simulink model "Noa_Nofusion_angle"  (R2020b)
settings: Solver=FixedStepDiscrete  StartTime=0.0  StopTime=Inf  FixedStep=0.01  RelTol=1e-3
PostLoadFcn:
  | if any(exist('dsrtsu_mdlpostloadfcn', 'file') ~= 0), dsrtsu_mdlpostloadfcn('Execute', bdroot); end
InitFcn:
  | , if any(exist('rtifpga_mdlclblib', 'file') ~= 0), rtifpga_mdlclblib('Init', bdroot); end,
  | , if any(exist('dsmpb_private', 'file') ~= 0), dsmpb_private('dsmpb_mdlclblib', 'Init', bdroot); end,
undefined symbols (not defined in the file): ACC_TimeGap_DecSetSwt, ACC_TimeGap_IncSetSwt, AccelPedalPosn, AccelPedalPosnVldty, AccelPedlPosnDiagc, AccPedalOverride, ACU_ShiftInProgress, ADAS_Posn_CurLane, AESSwtReq, ALC_SwtReq, BrkPedalSts, CC_ACC_CANCEL_OFFSwt, CC_ACC_CRUISE_OFFSwt, CC_ACC_DecSetSpd_SetSwt, CC_ACC_IncSetSpd_ResuSwt, CC_ACCSwtErr, CharSpd_ms, CSA_NODE, CURRENT_GEAR, CurrentGearValid, DiscIntNeverNeededParam, DrvDoorSts, DrvSBR, DrvTrqReqOvld, ECMACCInterface, ECMRespACC, ELKSwtReq, EngLimpHomeSts, EngSpd, EngState, EngState_PHEV, EngTrqMaxActSpd, EngTrqMinAct, EPS_DrvInpTrqVal_HighReslolution, EPS_FailSts, EPS_LKATorqOvrlDlvd, EPS_LKATorqOvrlDlvdVld, EPS_LKATrqOvlDlvdSts, EPS_SteerMod, EPS_TrqSnsrSts, EQ4_APPINFO, EQ4_LA_ELEM, EQ4_LA_HDR, EQ4_LAP_ELEM, EQ4_LAP_HDR, EQ4_LH_ELEM, EQ4_LH_HDR, EQ4_LRE_ELEM, EQ4_LRE_HDR, ESS_PedSwtReq, ESS_VehSwtReq, FFogLmpSts_F_Pbox, FLWheelDriveDirection, FLWheelSpd, FrntWiprSwtSts, FrntWshrSwtSts, FRWheelDriveDirection, FRWheelSpd, HazardLmpSwtSts, HCU_AccelPedalPosn_Diag ... (+151)
libraries: simulink x138, dsmpblib x33, canfdmsglib x10
(part 3 of 17)

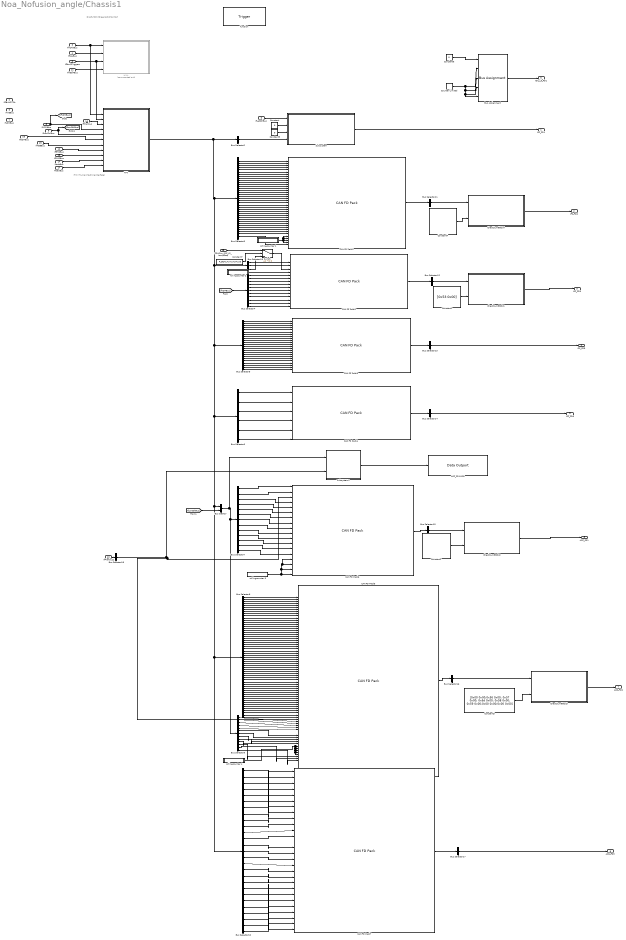
== system Noa_Nofusion_angle/Chassis1 ==
  note: DIAG-MON
      | (DiagnosticMonitor)
  note: HMI
      | (HumanMachineInterface)
  IfFaultTriggers : Inport
  IfFaultDTCs : Inport  Port=2
  IfVCANBus : Inport  Port=3  OutDataTypeStr=Bus: VCAN_BUS
  IfCALBus : Inport  Port=4
  IfVIEBus : Inport  Port=5
  IfVSMBus : Inport  Port=6
  IfLSMBus : Inport  Port=7
  IfLonCtrlBus : Inport  Port=8
  IfLatCtrlBus : Inport  Port=9
  IfPlanbus : Inport  Port=10
  IfVEQ4Bus : Inport  Port=11
  IfEHRBus : Inport  Port=12
  IfDMSBus : Inport  Port=13
  LaneBus : Inport  Port=14
  IfAEBBus : Inport  Port=15
  IfOSMBus : Inport  Port=16
  RoadBus : Inport  Port=17
  CSASim_IDC_L2_LampReq : Inport  Port=18
  function : TriggerPort  TriggerType=function-call  VariantControl=Variant
  ACC_FD1MSG : dsmpblib/Data Outport  Priority=-10000
      settings: SourceProductName=dSPACE Model Interface Blockset
  Bus Assignment : BusAssignment  AssignedSignals=RollingCounter_IDC_L3_1,RollingCounter_IDC_L3_3,RollingCounter_IDC_L3_5,RollingCounter_IDC_L3_4
  Bus Creator : BusCreator  Inputs=2
  Bus Selector10 : BusSelector  OutputSignals=HMI_ACC_FD4.ACCTgtObjAx,HMI_ACC_FD4.ACCTgtObjAy,HMI_ACC_FD4.ACCTgtObjCntAlive,HMI_ACC_FD4.ACCTgtObjDx,HMI_ACC_FD4.ACCTgtObjDy,HMI_ACC_FD4.ACCTgtObjExist,HMI_ACC_FD4.ACCTgtObjID,HMI_ACC_FD4.ACCTgtObjObstcl,HMI_ACC_FD4.ACCTgtObjState,HMI_ACC_FD4.ACCTgtObjVideoCfmd,HMI_ACC_FD4.ACCTgtObjVx,HMI_ACC_FD4.ACCTgtObjVy,HMI_ACC_FD4.ACC_SOSReq,HMI_ACC_FD4.BrdgDst,HMI_ACC_FD4.CurveDst,HMI_ACC_FD4.DrvgOnHiWay,HMI_ACC_FD4.DrvgOnRiLane,HMI_ACC_FD4.DrvrSts,HMI_ACC_FD4.HandsoffDetd,HMI_ACC_FD4.MapDataValid,HMI_ACC_FD4.NavSpdLimUnit,HMI_ACC_FD4.RampDst,HMI_ACC_FD4.RoadCrvt,HMI_ACC_FD4.RoadCrvtFar,HMI_ACC_FD4.SpdLimit,HMI_ACC_FD4.SpdLimitDst,HMI_ACC_FD4.TunnelDst
  Bus Selector{11..17} (7 alike) : BusSelector  OutputSignals=Data
  Bus Selector18 : BusSelector  OutputSignals=PLAN_Longctrl_DecelToStopReq
  Bus Selector19 : BusSelector  OutputSignals=HMI_IFC_FD3.IDC_L2_EmgyLightReq,HMI_IFC_FD3.IDC_L2_FWiperReq,HMI_IFC_FD3.IDC_L2_TurnLightReq
  Bus Selector2 : BusSelector  OutputSignals=IFCVibrationWarning
  Bus Selector3 : BusSelector  OutputSignals=AESErrSts,HMI_IFC_FD2.AESResp,HMI_IFC_FD2.AESSts,HMI_IFC_FD2.AESintervention,HMI_IFC_FD2.CameraBlockageSts,HMI_IFC_FD2.ELKMainState,HMI_IFC_FD2.ELKResp,ESSErrSts,HMI_IFC_FD2.ESSSts,HMI_IFC_FD2.ESS_PedResp,HMI_IFC_FD2.ESS_VehResp,HMI_IFC_FD2.ESSintervention,HMI_IFC_FD2.IFCCalibrationSts,HMI_IFC_FD2.IFCHUTInterface,HMI_IFC_FD2.IFC_Handsoffwarn,HMI_IFC_FD2.IFC_LaneCurve,HMI_IFC_FD2.IFC_LeLaneTyp,HMI_IFC_FD2.IFC_LeLane_dy,HMI_IFC_FD2.IFC_NextLeLaneTyp,HMI_IFC_FD2.IFC_NextLeLane_dy,HMI_IFC_FD2.IFC_NextRiLaneTyp,HMI_IFC_FD2.IFC_NextRiLane_dy,HMI_IFC_FD2.IFC_RiLaneTyp,HMI_IFC_FD2.IFC_RiLane_dy,HMI_IFC_FD2.IntelligentEvaResp,HMI_IFC_FD2.LCKResp,HMI_IFC_FD2.LDWResp,HMI_IFC_FD2.LDW_LKAWarn,HMI_IFC_FD2.LDW_LKA_Snvty,HMI_IFC_FD2.LKAResp,HMI_IFC_FD2.LSSErrSts,HMI_IFC_FD2.LSSFuncSts,HMI_IFC_FD2.LSSIntervention,HMI_IFC_FD2.LSSResp,HMI_IFC_FD2.LSSWarnFormResp,HMI_IFC_FD2.LaneAvailability,HMI_IFC_FD2.TJA_FollowSts
  Bus Selector4 : BusSelector  OutputSignals=VSM_TSR.TSRResp,VSM_TSR.TSRSpdLim,VSM_TSR.TSRSpdLimCfdc,VSM_TSR.TSRSpdLimSts,VSM_TSR.TSRSpdLimUnit,VSM_TSR.TSRSpdLimWarn,VSM_TSR.TSRSts,VSM_TSR.TSRTrfcSignVal,VSM_TSR.TSRTrfcSignValCfdc,VSM_TSR.TSRWarnResp,VSM_TSR.TSR_Snvty
  Bus Selector5 : BusSelector  OutputSignals=HMI_IFC_FD5.IFC_Line01_Curv,HMI_IFC_FD5.IFC_Line01_CurvChange,HMI_IFC_FD5.IFC_Line01_Dy,HMI_IFC_FD5.IFC_Line01_Type,HMI_IFC_FD5.IFC_Line02_Curv,HMI_IFC_FD5.IFC_Line02_CurvChange,HMI_IFC_FD5.IFC_Line02_Dy,HMI_IFC_FD5.IFC_Line02_Type,HMI_IFC_FD5.IFC_Line03_Curv,HMI_IFC_FD5.IFC_Line03_CurvChange,HMI_IFC_FD5.IFC_Line03_Dy,HMI_IFC_FD5.IFC_Line03_Type,HMI_IFC_FD5.IFC_Line04_Curv,HMI_IFC_FD5.IFC_Line04_CurvChange,HMI_IFC_FD5.IFC_Line04_Dy,HMI_IFC_FD5.IFC_Line04_Type,HMI_IFC_FD5.IFC_Roadedge01_Curv,HMI_IFC_FD5.IFC_Roadedge01_CurvChange,HMI_IFC_FD5.IFC_Roadedge01_Dy,HMI_IFC_FD5.IFC_Roadedge01_Type,HMI_IFC_FD5.IFC_Roadedge02_Curv,HMI_IFC_FD5.IFC_Roadedge02_CurvChange,HMI_IFC_FD5.IFC_Roadedge02_Dy,HMI_IFC_FD5.IFC_Roadedge02_Type
  Bus Selector6 : BusSelector  OutputSignals=HMI_IFC_FD6.IFC_Line01_HeadingAngle,HMI_IFC_FD6.IFC_Line02_HeadingAngle,HMI_IFC_FD6.IFC_Line03_HeadingAngle,HMI_IFC_FD6.IFC_Line04_HeadingAngle,HMI_IFC_FD6.IFC_Roadedge01_HeadingAngle,HMI_IFC_FD6.IFC_Roadedge02_HeadingAngle
  Bus Selector7 : BusSelector  OutputSignals=HMI.HMI_ACC_FD1.ACC_CRInterface,HMI.HMI_ACC_FD1.ActualTargetSpeed,signal2.LONC_CTRL_OUT.Longctrl_Decel_Req,signal2.LONC_CTRL_OUT.Longctrl_Decel_ReqValue,HMI.HMI_ACC_FD1.Longctrl_DrvOFF_Req,signal2.LONC_CTRL_OUT.Longctrl_EngTrqReq,signal2.LONC_CTRL_OUT.Longctrl_EngTrqReqActive,HMI.HMI_ACC_FD1.Longctrl_FuelCutOffPrevn,signal2.LONC_Hybrid_CTRL_OUT.Longctrl_HCUTrqReq,signal2.LONC_Hybrid_CTRL_OUT.Longctrl_HCUTrqReqActive,HMI.HMI_ACC_FD1.Longctrl_ModSts,HMI.HMI_ACC_FD1.Longctrl_ParkShiftReq,HMI.HMI_ACC_FD1.Longctrl_VehHldReq
  Bus Selector8 : BusSelector  OutputSignals=HMI_ACC_FD2.ACC_EgoStatus,HMI_ACC_FD2.ACC_FctSts,HMI_ACC_FD2.ACC_InterSysInfoDisp,HMI_ACC_FD2.ACC_LeTargrtDection,HMI_ACC_FD2.ACC_LeTargrt_02_Detn,HMI_ACC_FD2.ACC_LeTgtDx,HMI_ACC_FD2.ACC_LeTgtDy,HMI_ACC_FD2.ACC_LeTgtHeading,HMI_ACC_FD2.ACC_LeTgtObjBarDisp,HMI_ACC_FD2.ACC_LeTgtTyp,HMI_ACC_FD2.ACC_LeTgt_02_Dy,HMI_ACC_FD2.ACC_LeTgt_02_Dx,HMI_ACC_FD2.ACC_LeTgt_02_Typ,HMI_ACC_FD2.ACC_LeTgtfusion,HMI_ACC_FD2.ACC_ModDisp,HMI_ACC_FD2.ACC_ObjDetecte,HMI_ACC_FD2.ACC_PotentialTgtDetn,HMI_ACC_FD2.ACC_PotentialTgtDx,HMI_ACC_FD2.ACC_PotentialTgtDy,HMI_ACC_FD2.ACC_PotentialTgtHeading,HMI_ACC_FD2.ACC_PotentialTgtTyp,HMI_ACC_FD2.ACC_PotentialTgtfusion,HMI_ACC_FD2.ACC_RiTargrtDetn,HMI_ACC_FD2.ACC_RiTargrt_02_Detn,HMI_ACC_FD2.ACC_RiTgtDx,HMI_ACC_FD2.ACC_RiTgtDy,HMI_ACC_FD2.ACC_RiTgtHeading,HMI_ACC_FD2.ACC_RiTgtObjBarDisp,HMI_ACC_FD2.ACC_RiTgtTyp,HMI_ACC_FD2.ACC_RiTgt_02_Dx,HMI_ACC_FD2.ACC_RiTgt_02_Dy,HMI_ACC_FD2.ACC_RiTgt_02_Typ,HMI_ACC_FD2.ACC_RiTgtfusion,HMI_ACC_FD2.ACC_RlvTgtDetn,HMI_ACC_FD2.ACC_RlvTgtDx,HMI_ACC_FD2.ACC_RlvTgtDy,HMI_ACC_FD2.ACC_RlvTgtHeading,HMI_ACC_FD2.ACC_RlvTgtTyp,HMI_ACC_FD2.ACC_RlvTgtfusion,HMI_ACC_FD2.ACC_SpdSetValue,HMI_ACC_FD2.ACC_TakeOverReq,HMI_ACC_FD2.ACC_TgtObjBarDisp,HMI_ACC_FD2.ACC_TimeGapSet,HMI_ACC_FD2.ADAS_DriverInloop_Monitor,HMI_ACC_FD2.ALC_InterSysInfoDisp,HMI_ACC_FD2.ALC_Resp,HMI_ACC_FD2.CruCha_ModDisp,HMI_ACC_FD2.CruChar_InterSysInfoDisp,HMI_ACC_FD2.HWA_InterSysInfoDisp,HMI_ACC_FD2.HWA_LaneChange,HMI_ACC_FD2.HWA_LaneChangeReq,HMI_ACC_FD2.HWA_ModDisp,HMI_ACC_FD2.HWA_Resp,HMI_ACC_FD2.HWA_SnvtySet_Resp,HMI_ACC_FD2.HWA_warning,HMI_ACC_FD2.ICA_HandsOffResp,HMI_ACC_FD2.ISL_InterSysInfoDisp,HMI_ACC_FD2.ISL_Resp,HMI_ACC_FD2.IntelligentCurveAct
  Bus Selector9 : BusSelector  OutputSignals=signal2.LONC_CTRL_OUT.Longctrl_Decel_ReqValue,signal2.LONC_CTRL_OUT.Longctrl_Decel_Req,HMI.HMI_ACC_FD1.Longctrl_DrvOFF_Req,signal2.LONC_CTRL_OUT.Longctrl_EngTrqReqActive,signal2.LONC_CTRL_OUT.Longctrl_EngTrqReq,HMI.HMI_ACC_FD2.Longctrl_HazActv,HMI.HMI_ACC_FD2.Longctrl_ModSts_DVR,HMI.HMI_ACC_FD2.Longctrl_ParkShiftReq_DVR,HMI.HMI_ACC_FD2.Longctrl_VehHldReq_DVR,HMI.HMI_ACC_FD2.Request_driveoff,HMI.HMI_ACC_FD2.TJA_ACC_SelSts,HMI.HMI_ACC_FD2.TJA_ICA_InterSysInfoDisp,HMI.HMI_ACC_FD2.TJA_ICA_ModDisp
  CAN FD Pack1 : canfdmsglib/CAN FD Pack  MsgList=(none)  MsgName=IFC_FD2  ProtocolMode=CAN FD  MsgIDType=Standard (11-bit identifier)  MsgIdentifier=573  MsgLength=64  Remote=off  BRSSwitch=on  ApplyMinMax=off  SignalInfo={ 'AESErrSts', '93', '1', 'BE', 'unsigned', 'Standard', '0', '1', '0', '0', '1'; 'AESResp', '75', '1', 'BE', 'unsigned', 'Standard', '0', '1', '0', '0', '1'; 'AESSts', '80', '2', 'BE', 'unsigned', 'Standard', '0', '1', '0', '0', '3'; 'AESintervention', '90', '2', 'BE', 'unsigned', 'Standard', '0', '1', '0', '0', '3'; 'CameraBlockageSts', '152', '1', 'BE', 'unsigned', 'Standard', '0', '1', '0', '0', '1'; 'ELKMainState', '149', '3', 'BE', 'unsigned', 'Standard', '0', '1', '0', '0', '7'; 'ELKResp', '76', '1', 'BE', 'unsigned', 'Standard', '0', '1', '0', '0', '1'; 'ESSErrSts', '92', '1', 'BE', 'unsigned', 'Standard', '0', '1', '0', '0', '1'; 'ESSSts', '94', '2', 'BE', 'unsigned', 'Standard', '0', '1', '0', '0', '3'; 'ESS_PedResp', '87', '1', 'BE', 'unsigned', 'Standard', '0', '1', '0', '0', '1'; 'ESS_VehResp', '86', '1', 'BE', 'unsigned', 'Standard', '0', '1', '0', '0', '1'; 'ESSintervention', '88', '2', 'BE', 'unsigned', 'Standard', '0', '1', '0', '0', '3'; 'IFCCalibrationSts', '153', '2', 'BE', 'unsigned', 'Standard', '0', '1', '0', '0', '3'; 'IFCHUTInterface', '72', '1', 'BE', 'unsigned', 'Standard', '0', '1', '0', '0', '1'; 'IFC_Handsoffwarn', '155', '3', 'BE', 'unsigned', 'Standard', '0', '1', '0', '0', '7'; 'IFC_LaneCurve', '212', '12', 'BE', 'unsigned', 'Standard', '0', '1.5e-05', '-0.030705', '-0.030705', '0.030705'; 'IFC_LeLaneTyp', '209', '3', 'BE', 'unsigned', 'Standard', '0', '1', '0', '0', '7'; 'IFC_LeLane_dy', '236', '12', 'BE', 'unsigned', 'Standard', '0', '0.0039063', '-8', '-8', '7.9922'; 'IFC_NextLeLaneTyp', '219', '3', 'BE', 'unsigned', 'Standard', '0', '1', '0', '0', '7'; 'IFC_NextLeLane_dy', '276', '12', 'BE', 'unsigned', 'Standard', '0', '0.0039063', '-8', '-8', '7.9922'; 'IFC_NextRiLaneTyp', '216', '3', 'BE', 'unsigned', 'Standard', '0', '1', '0', '0', '7'; 'IFC_NextRiLane_dy', '280', '12', 'BE', 'unsigned', 'Standard', '0', '0.0039063', '-8', '-8', '7.9922'; 'IFC_RiLaneTyp', '222', '3', 'BE', 'unsigned', 'Standard', '0', '1', '0', '0', '7'; 'IFC_RiLane_dy', '240', '12', 'BE', 'unsigned', 'Standard', '0', '0.0039063', '-8', '-8', '7.9922'; 'IntelligentEvaResp', '82', '1', 'BE', 'unsigned', 'Standard', '0', '1', '0', '0', '1'; 'LCKResp', '77', '1', 'BE', 'unsigned', 'Standard', '0', '1', '0', '0', '1'; 'LDWResp', '79', '1', 'BE', 'unsigned', 'Standard', '0', '1', '0', '0', '1'; 'LDW_LKAWarn', '142', '2', 'BE', 'unsigned', 'Standard', '0', '1', '0', '0', '3'; 'LDW_LKA_Snvty', '73', '2', 'BE', 'unsigned', 'Standard', '0', '1', '0', '0', '3'; 'LKAResp', '78', '1', 'BE', 'unsigned', 'Standard', '0', '1', '0', '0', '1'; 'LSSErrSts', '158', '3', 'BE', 'unsigned', 'Standard', '0', '1', '0', '0', '7'; 'LSSFuncSts', '136', '3', 'BE', 'unsigned', 'Standard', '0', '1', '0', '0', '7'; 'LSSIntervention', '139', '3', 'BE', 'unsigned', 'Standard', '0', '1', '0', '0', '7'; 'LSSResp', '83', '1', 'BE', 'unsigned', 'Standard', '0', '1', '0', '0', '1'; 'LSSWarnFormResp', '84', '2', 'BE', 'unsigned', 'Standard', '0', '1', '0', '0', '3'; 'LaneAvailability', '147', '2', 'BE', 'unsigned', 'Standard', '0', '1', '0', '0', '3'; 'RollingCounter_IFC3', '120', '4', 'BE', 'unsigned', 'Standard', '0', '1', '0', '0', '15'; 'RollingCounter_IFC4', '184', '4', 'BE', 'unsigned', 'Standard', '0', '1', '0', '0', '15'; 'RollingCounter_IFC5', '248', '4', 'BE', 'unsigned', 'Standard', '0', '1', '0', '0', '15'; 'RollingCounter_IFC6', '312', '4', 'BE', 'unsigned', 'Standard', '0', '1', '0', '0', '15'; 'TJA_FollowSts', '145', '2', 'BE', 'unsigned', 'Standard', '0', '1', '0', '0', '3' }
      settings: SourceProductBaseCode=VN  DataFormat=manually specified signals
  CAN FD Pack2 : canfdmsglib/CAN FD Pack  MsgList=(none)  MsgName=IFC_FD3  ProtocolMode=CAN FD  MsgIDType=Standard (11-bit identifier)  MsgIdentifier=719  MsgLength=64  Remote=off  BRSSwitch=on  ApplyMinMax=off  SignalInfo={ 'HMA_HibeamReq', '112', '2', 'BE', 'unsigned', 'Standard', '0', '1', '0', '0', '3'; 'HMA_Sts', '125', '3', 'BE', 'unsigned', 'Standard', '0', '1', '0', '0', '7'; 'IDC_L2_EmgyLightReq', '111', '1', 'BE', 'unsigned', 'Standard', '0', '1', '0', '0', '1'; 'IDC_L2_FWiperReq', '105', '3', 'BE', 'unsigned', 'Standard', '0', '1', '0', '0', '7'; 'IDC_L2_TurnLightReq', '109', '2', 'BE', 'unsigned', 'Standard', '0', '1', '0', '0', '3'; 'RollingCounter_IFC7', '120', '4', 'BE', 'unsigned', 'Standard', '0', '1', '0', '0', '15'; 'TSRResp', '79', '1', 'BE', 'unsigned', 'Standard', '0', '1', '0', '0', '1'; 'TSRSpdLim', '82', '6', 'BE', 'unsigned', 'Standard', '0', '1', '0', '0', '63'; 'TSRSpdLimCfdc', '75', '2', 'BE', 'unsigned', 'Standard', '0', '1', '0', '0', '3'; 'TSRSpdLimSts', '80', '2', 'BE', 'unsigned', 'Standard', '0', '1', '0', '0', '3'; 'TSRSpdLimUnit', '77', '2', 'BE', 'unsigned', 'Standard', '0', '1', '0', '0', '3'; 'TSRSpdLimWarn', '101', '1', 'BE', 'unsigned', 'Standard', '0', '1', '0', '0', '1'; 'TSRSts', '72', '3', 'BE', 'unsigned', 'Standard', '0', '1', '0', '0', '7'; 'TSRTrfcSignVal', '102', '8', 'BE', 'unsigned', 'Standard', '0', '1', '0', '0', '255'; 'TSRTrfcSignValCfdc', '94', '2', 'BE', 'unsigned', 'Standard', '0', '1', '0', '0', '3'; 'TSRWarnResp', '108', '1', 'BE', 'unsigned', 'Standard', '0', '1', '0', '0', '1'; 'TSR_Snvty', '96', '5', 'BE', 'unsigned', 'Standard', '0', '1', '-15', '-15', '15' }
      settings: SourceProductBaseCode=VN  DataFormat=manually specified signals
  CAN FD Pack3 : canfdmsglib/CAN FD Pack  CANdbFile=C:\Users\GW00133806\Desktop\LC\V61_APE_HWA\dbc\V71_ADCAN.dbc  MsgList=(none)  MsgName=IFC_FD5  ProtocolMode=CAN FD  MsgIDType=Standard (11-bit identifier)  MsgIdentifier=415  MsgLength=64  Remote=off  BRSSwitch=on  ApplyMinMax=off  SignalInfo={'IFC_Line01_Curv','36','15','BE','unsigned','Standard','0','1.6e-05','-0.25','-0.25','0.25';'IFC_Line01_CurvChange','48','20','BE','unsigned','Standard','0','5e-08','-0.024','-0.024','0.024';'IFC_Line01_Dy','19','13','BE','unsigned','Standard','0','0.01','-30','-30','30';'IFC_Line01_Type','60','4','BE','unsigned','Standard','0','1','0','0','15';'IFC_Line02_Curv','100','15','BE','unsigned','Standard','0','1.6e-05','-0.25','-0.25','0.25';'IFC_Line02_CurvChange','112','20','BE','unsigned','Standard','0','5e-08','-0.024','-0.024','0.024';'IFC_Line02_Dy','83','13','BE','unsigned','Standard','0','0.01','-30','-30','30';'IFC_Line02_Type','124','4','BE','unsigned','Standard','0','1','0','0','15';'IFC_Line03_Curv','164','15','BE','unsigned','Standard','0','1.6e-05','-0.25','-0.25','0.25';'IFC_Line03_CurvChange','176','20','BE','unsigned','Standard','0','5e-08','-0.024','-0.024','0.024';'IFC_Line03_Dy','147','13','BE','unsigned','Standard','0','0.01','-30','-30','30';'IFC_Line03_Type','188','4','BE','unsigned','Standard','0','1','0','0','15';'IFC_Line04_Curv','228','15','BE','unsigned','Standard','0','1.6e-05','-0.25','-0.25','0.25';'IFC_Line04_CurvChange','240','20','BE','unsigned','Standard','0','5e-08','-0.024','-0.024','0.024';'IFC_Line04_Dy','211','13','BE','unsigned','Standard','0','0.01','-30','-30','30';'IFC_Line04_Type','252','4','BE','unsigned','Standard','0','1','0','0','15';'IFC_Roadedge01_Curv','292','15','BE','unsigned','Standard','0','1.6e-05','-0.25','-0.25','0.25';'IFC_Roadedge01_CurvChange','304','20','BE','unsigned','Standard','0','5e-08','-0.024','-0.024','0.024';'IFC_Roadedge01_Dy','275','13','BE','unsigned','Standard','0','0.01','-30','-30','30';'IFC_Roadedge01_Type','316','4','BE','unsigned','Standard','0','1','0','0','15';'IFC_Roadedge02_Curv','356','15','BE','unsigned','Standard','0','1.6e-05','-0.25','-0.25','0.25';'IFC_Roadedge02_CurvChange','368','20','BE','unsigned','Standard','0','5e-08','-0.024','-0.024','0.024';'IFC_Roadedge02_Dy','339','13','BE','unsigned','Standard','0','0.01','-30','-30','30';'IFC_Roadedge02_Type','380','4','BE','unsigned','Standard','0','1','0','0','15'}
      settings: SourceProductBaseCode=VN  DataFormat=CANdb specified signals
  CAN FD Pack4 : canfdmsglib/CAN FD Pack  CANdbFile=C:\Users\GW00133806\Desktop\LC\V61_APE_HWA\dbc\V71_ADCAN.dbc  MsgList=(none)  MsgName=IFC_FD6  ProtocolMode=CAN FD  MsgIDType=Standard (11-bit identifier)  MsgIdentifier=546  MsgLength=64  Remote=off  BRSSwitch=on  ApplyMinMax=off  SignalInfo={'IFC_Line01_DxEnd','34','15','BE','unsigned','Standard','0','0.01','0','0','200';'IFC_Line01_DxStart','17','15','BE','unsigned','Standard','0','0.01','0','0','200';'IFC_Line01_HeadingAngle','41','9','BE','unsigned','Standard','0','0.01','-2','-2','2';'IFC_Line02_DxEnd','97','15','BE','unsigned','Standard','0','0.01','0','0','200';'IFC_Line02_DxStart','81','15','BE','unsigned','Standard','0','0.01','0','0','200';'IFC_Line02_HeadingAngle','48','9','BE','unsigned','Standard','0','0.01','-2','-2','2';'IFC_Line03_DxEnd','145','15','BE','unsigned','Standard','0','0.01','0','0','200';'IFC_Line03_DxStart','113','15','BE','unsigned','Standard','0','0.01','0','0','200';'IFC_Line03_HeadingAngle','152','9','BE','unsigned','Standard','0','0.01','-2','-2','2';'IFC_Line04_DxEnd','209','15','BE','unsigned','Standard','0','0.01','0','0','200';'IFC_Line04_DxStart','169','15','BE','unsigned','Standard','0','0.01','0','0','200';'IFC_Line04_HeadingAngle','176','9','BE','unsigned','Standard','0','0.01','-2','-2','2';'IFC_Roadedge01_DxEnd','241','15','BE','unsigned','Standard','0','0.01','0','0','200';'IFC_Roadedge01_DxStart','225','15','BE','unsigned','Standard','0','0.01','0','0','200';'IFC_Roadedge01_HeadingAngle','279','9','BE','unsigned','Standard','0','0.01','-2','-2','2';'IFC_Roadedge02_DxEnd','297','15','BE','unsigned','Standard','0','0.01','0','0','200';'IFC_Roadedge02_DxStart','280','15','BE','unsigned','Standard','0','0.01','0','0','200';'IFC_Roadedge02_HeadingAngle','304','9','BE','unsigned','Standard','0','0.01','-2','-2','2'}
      settings: SourceProductBaseCode=VN  DataFormat=CANdb specified signals
  CAN FD Pack5 : canfdmsglib/CAN FD Pack  MsgList=(none)  MsgName=ACC_FD2  ProtocolMode=CAN FD  MsgIDType=Standard (11-bit identifier)  MsgIdentifier=683  MsgLength=64  Remote=off  BRSSwitch=on  ApplyMinMax=off  SignalInfo={ 'ACC_EgoStatus', '283', '2', 'BE', 'unsigned', 'Standard', '0', '1', '0', '0', '3'; 'ACC_FctSts', '145', '2', 'BE', 'unsigned', 'Standard', '0', '1', '0', '0', '3'; 'ACC_InterSysInfoDisp', '137', '5', 'BE', 'unsigned', 'Standard', '0', '1', '0', '0', '31'; 'ACC_LeTargrtDection', '346', '2', 'BE', 'unsigned', 'Standard', '0', '1', '0', '0', '3'; 'ACC_LeTargrt_02_Detn', '27', '2', 'BE', 'unsigned', 'Standard', '0', '1', '0', '0', '3'; 'ACC_LeTgtDx', '351', '9', 'BE', 'unsigned', 'Standard', '0', '0.5', '0', '0', '150'; 'ACC_LeTgtDy', '328', '8', 'BE', 'unsigned', 'Standard', '0', '0.1', '-8', '-8', '8'; 'ACC_LeTgtHeading', '402', '6', 'BE', 'unsigned', 'Standard', '0', '0.05', '-1.5', '-1.5', '1.5'; 'ACC_LeTgtObjBarDisp', '45', '3', 'BE', 'unsigned', 'Standard', '0', '1', '0', '0', '7'; 'ACC_LeTgtTyp', '348', '3', 'BE', 'unsigned', 'Standard', '0', '1', '0', '0', '7'; 'ACC_LeTgt_02_Dx', '16', '9', 'BE', 'unsigned', 'Standard', '0', '0.5', '0', '0', '150'; 'ACC_LeTgt_02_Dy', '9', '7', 'BE', 'unsigned', 'Standard', '0', '0.1', '0', '0', '8'; 'ACC_LeTgt_02_Typ', '29', '3', 'BE', 'unsigned', 'Standard', '0', '1', '0', '0', '7'; 'ACC_LeTgtfusion', '392', '1', 'BE', 'unsigned', 'Standard', '0', '1', '0', '0', '1'; 'ACC_ModDisp', '147', '5', 'BE', 'unsigned', 'Standard', '0', '1', '0', '0', '31'; 'ACC_ObjDetecte', '143', '1', 'BE', 'unsigned', 'Standard', '0', '1', '0', '0', '1'; 'ACC_PotentialTgtDetn', '308', '2', 'BE', 'unsigned', 'Standard', '0', '1', '0', '0', '3'; 'ACC_PotentialTgtDx', '287', '9', 'BE', 'unsigned', 'Standard', '0', '0.5', '0', '0', '150'; 'ACC_PotentialTgtDy', '264', '8', 'BE', 'unsigned', 'Standard', '0', '0.1', '-8', '-8', '8'; 'ACC_PotentialTgtHeading', '420', '6', 'BE', 'unsigned', 'Standard', '0', '0.05', '-1.5', '-1.5', '1.5'; 'ACC_PotentialTgtTyp', '305', '3', 'BE', 'unsigned', 'Standard', '0', '1', '0', '0', '7'; 'ACC_PotentialTgtfusion', '400', '1', 'BE', 'unsigned', 'Standard', '0', '1', '0', '0', '1'; 'ACC_RiTargrtDetn', '344', '2', 'BE', 'unsigned', 'Standard', '0', '1', '0', '0', '3'; 'ACC_RiTargrt_02_Detn', '25', '2', 'BE', 'unsigned', 'Standard', '0', '1', '0', '0', '3'; 'ACC_RiTgtDx', '375', '9', 'BE', 'unsigned', 'Standard', '0', '0.5', '0', '0', '150'; 'ACC_RiTgtDy', '352', '8', 'BE', 'unsigned', 'Standard', '0', '0.1', '-8', '-8', '8'; 'ACC_RiTgtHeading', '410', '6', 'BE', 'unsigned', 'Standard', '0', '0.05', '-1.5', '-1.5', '1.5'; 'ACC_RiTgtObjBarDisp', '42', '3', 'BE', 'unsigned', 'Standard', '0', '1', '0', '0', '7'; 'ACC_RiTgtTyp', '372', '3', 'BE', 'unsigned', 'Standard', '0', '1', '0', '0', '7'; 'ACC_RiTgt_02_Dx', '32', '9', 'BE', 'unsigned', 'Standard', '0', '0.5', '0', '0', '150'; 'ACC_RiTgt_02_Dy', '49', '7', 'BE', 'unsigned', 'Standard', '0', '0.1', '-8', '-8', '0'; 'ACC_RiTgt_02_Typ', '61', '3', 'BE', 'unsigned', 'Standard', '0', '1', '0', '0', '7'; 'ACC_RiTgtfusion', '401', '1', 'BE', 'unsigned', 'Standard', '0', '1', '0', '0', '1'; 'ACC_RlvTgtDetn', '285', '2', 'BE', 'unsigned', 'Standard', '0', '1', '0', '0', '3'; 'ACC_RlvTgtDx', '311', '9', 'BE', 'unsigned', 'Standard', '0', '0.5', '0', '0', '150'; 'ACC_RlvTgtDy', '288', '8', 'BE', 'unsigned', 'Standard', '0', '0.1', '-8', '-8', '8'; 'ACC_RlvTgtHeading', '393', '6', 'BE', 'unsigned', 'Standard', '0', '0.05', '-1.5', '-1.5', '1.5'; 'ACC_RlvTgtTyp', '280', '3', 'BE', 'unsigned', 'Standard', '0', '1', '0', '0', '7'; 'ACC_RlvTgtfusion', '399', '1', 'BE', 'unsigned', 'Standard', '0', '1', '0', '0', '1'; 'ACC_SpdSetValue', '176', '8', 'BE', 'unsigned', 'Standard', '0', '1', '0', '0', '255'; 'ACC_TakeOverReq', '142', '1', 'BE', 'unsigned', 'Standard', '0', '1', '0', '0', '1'; 'ACC_TgtObjBarDisp', '157', '3', 'BE', 'unsigned', 'Standard', '0', '1', '0', '0', '7'; 'ACC_TimeGapSet', '168', '3', 'BE', 'unsigned', 'Standard', '0', '1', '0', '0', '7'; 'ADAS_DriverInloop_Monitor', '209', '3', 'BE', 'unsigned', 'Standard', '0', '1', '7', '7', '7'; 'ALC_InterSysInfoDisp', '126', '2', 'BE', 'unsigned', 'Standard', '0', '1', '0', '0', '3'; 'ALC_Resp', '73', '1', 'BE', 'unsigned', 'Standard', '0', '1', '0', '0', '1'; 'CruCha_ModDisp', '164', '4', 'BE', 'unsigned', 'Standard', '0', '1', '0', '0', '15'; 'CruChar_InterSysInfoDisp', '188', '4', 'BE', 'unsigned', 'Standard', '0', '1', '0', '0', '15'; 'HWA_InterSysInfoDisp', '200', '4', 'BE', 'unsigned', 'Standard', '0', '1', '0', '0', '15'; 'HWA_LaneChange', '212', '2', 'BE', 'unsigned', 'Standard', '0', '1', '0', '0', '3'; 'HWA_LaneChangeReq', '221', '3', 'BE', 'unsigned', 'Standard', '0', '1', '0', '0', '7'; 'HWA_ModDisp', '204', '4', 'BE', 'unsigned', 'Standard', '0', '1', '0', '0', '15'; 'HWA_Resp', '77', '1', 'BE', 'unsigned', 'Standard', '0', '1', '0', '0', '1'; 'HWA_SnvtySet_Resp', '75', '2', 'BE', 'unsigned', 'Standard', '0', '1', '0', '0', '3'; 'HWA_warning', '216', '2', 'BE', 'unsigned', 'Standard', '0', '1', '0', '0', '3'; 'ICA_HandsOffResp', '78', '1', 'BE', 'unsigned', 'Standard', '0', '1', '0', '0', '1'; 'ISL_InterSysInfoDisp', '171', '2', 'BE', 'unsigned', 'Standard', '0', '1', '0', '0', '3'; 'ISL_Resp', '79', '1', 'BE', 'unsigned', 'Standard', '0', '1', '0', '0', '1'; 'IntelligentCurveAct', '319', '1', 'BE', 'unsigned', 'Standard', '0', '1', '0', '0', '1'; 'Longctrl_DecelToStopReq_DVR', '119', '1', 'BE', 'unsigned', 'Standard', '0', '1', '0', '0', '1'; 'Longctrl_Decel_ReqValue_DVR', '104', '8', 'BE', 'unsigned', 'Standard', '0', '0.05', '-7', '-7', '5.75'; 'Longctrl_Decel_Req_DVR', '81', '1', 'BE', 'unsigned', 'Standard', '0', '1', '0', '0', '1'; 'Longctrl_DrvOFF_Req_DVR', '86', '1', 'BE', 'unsigned', 'Standard', '0', '1', '0', '0', '1'; 'Longctrl_EngTrqReqActive_DVR', '80', '1', 'BE', 'unsigned', 'Standard', '0', '1', '0', '0', '1'; 'Longctrl_EngTrqReq_DVR', '96', '16', 'BE', 'unsigned', 'Standard', '0', '0.0030518', '-100', '-100', '99.9997'; 'Longctrl_HCUTrqReqActive_DVR', '116', '1', 'BE', 'unsigned', 'Standard', '0', '1', '0', '0', '1'; 'Longctrl_HCUTrqReq_DVR', '232', '16', 'BE', 'unsigned', 'Standard', '0', '0.5', '-16384', '-16384', '16383.5'; 'Longctrl_HazActv', '155', '2', 'BE', 'unsigned', 'Standard', '0', '1', '0', '0', '3'; 'Longctrl_ModSts_DVR', '82', '4', 'BE', 'unsigned', 'Standard', '0', '1', '0', '0', '15'; 'Longctrl_ParkShiftReq_DVR', '117', '2', 'BE', 'unsigned', 'Standard', '0', '1', '0', '0', '3'; 'Longctrl_VehHldReq_DVR', '87', '1', 'BE', 'unsigned', 'Standard', '0', '1', '0', '0', '1'; 'Request_driveoff', '381', '3', 'BE', 'unsigned', 'Standard', '0', '1', '0', '0', '7'; 'RollingCounter_ACC3', '120', '4', 'BE', 'unsigned', 'Standard', '0', '1', '0', '0', '15'; 'RollingCounter_ACC4', '184', '4', 'BE', 'unsigned', 'Standard', '0', '1', '0', '0', '15'; 'RollingCounter_ACC6', '312', '4', 'BE', 'unsigned', 'Standard', '0', '1', '0', '0', '15'; 'RollingCounter_ACC7', '376', '4', 'BE', 'unsigned', 'Standard', '0', '1', '0', '0', '15'; 'RollingCounter_ACC8', '248', '4', 'BE', 'unsigned', 'Standard', '0', '1', '0', '0', '15'; 'TJA_ACC_SelSts', '152', '3', 'BE', 'unsigned', 'Standard', '0', '1', '0', '0', '7'; 'TJA_ICA_InterSysInfoDisp', '161', '3', 'BE', 'unsigned', 'Standard', '0', '1', '0', '0', '7'; 'TJA_ICA_ModDisp', '173', '3', 'BE', 'unsigned', 'Standard', '0', '1', '0', '0', '7'; 'TargetCutinPro', '430', '6', 'BE', 'unsigned', 'Standard', '0', '0.02', '0', '0', '1'; 'TargetCutoutPro', '424', '6', 'BE', 'unsigned', 'Standard', '0', '0.02', '0', '0', '1' }
      settings: SourceProductBaseCode=VN  DataFormat=manually specified signals
  CAN FD Pack6 : canfdmsglib/CAN FD Pack  MsgList=(none)  MsgName=ACC_FD1  ProtocolMode=CAN FD  MsgIDType=Standard (11-bit identifier)  MsgIdentifier=323  MsgLength=64  Remote=off  BRSSwitch=on  ApplyMinMax=off  SignalInfo={ 'ACC_CRInterface', '191', '1', 'BE', 'unsigned', 'Standard', '0', '1', '0', '0', '1'; 'ActualTargetSpeed', '112', '8', 'BE', 'unsigned', 'Standard', '0', '1', '0', '0', '254'; 'Longctrl_DecelToStopReq', '101', '1', 'BE', 'unsigned', 'Standard', '0', '1', '0', '0', '1'; 'Longctrl_Decel_Req', '72', '1', 'BE', 'unsigned', 'Standard', '0', '1', '0', '0', '1'; 'Longctrl_Decel_ReqValue', '104', '8', 'BE', 'unsigned', 'Standard', '0', '0.05', '-7', '-7', '5.75'; 'Longctrl_DrvOFF_Req', '78', '1', 'BE', 'unsigned', 'Standard', '0', '1', '0', '0', '1'; 'Longctrl_EngTrqReq', '88', '16', 'BE', 'unsigned', 'Standard', '0', '0.0030518', '-100', '-100', '99.9997'; 'Longctrl_EngTrqReqActive', '103', '1', 'BE', 'unsigned', 'Standard', '0', '1', '0', '0', '1'; 'Longctrl_FuelCutOffPrevn', '102', '1', 'BE', 'unsigned', 'Standard', '0', '1', '0', '0', '1'; 'Longctrl_HCUTrqReq', '224', '16', 'BE', 'unsigned', 'Standard', '0', '0.5', '-16384', '-16384', '16383.5'; 'Longctrl_HCUTrqReqActive', '239', '1', 'BE', 'unsigned', 'Standard', '0', '1', '0', '0', '1'; 'Longctrl_ModSts', '74', '4', 'BE', 'unsigned', 'Standard', '0', '1', '0', '0', '15'; 'Longctrl_ParkShiftReq', '98', '2', 'BE', 'unsigned', 'Standard', '0', '1', '0', '0', '3'; 'Longctrl_VehHldReq', '79', '1', 'BE', 'unsigned', 'Standard', '0', '1', '0', '0', '1'; 'RollingCounter_ACC1', '120', '4', 'BE', 'unsigned', 'Standard', '0', '1', '0', '0', '15'; 'RollingCounter_ACC10', '248', '4', 'BE', 'unsigned', 'Standard', '0', '1', '0', '0', '15'; 'RollingCounter_ACC11', '56', '4', 'BE', 'unsigned', 'Standard', '0', '1', '0', '0', '15'; 'RollingCounter_ACC2', '184', '4', 'BE', 'unsigned', 'Standard', '0', '1', '0', '0', '15' }
      settings: SourceProductBaseCode=VN  DataFormat=manually specified signals
  CAN FD Pack7 : canfdmsglib/CAN FD Pack  MsgList=(none)  MsgName=ACC_FD4  ProtocolMode=CAN FD  MsgIDType=Standard (11-bit identifier)  MsgIdentifier=696  MsgLength=64  Remote=off  BRSSwitch=on  ApplyMinMax=off  SignalInfo={ 'ACCTgtObjAx', '370', '10', 'BE', 'unsigned', 'Standard', '0', '0.03125', '-16', '-16', '15.9688'; 'ACCTgtObjAy', '376', '10', 'BE', 'unsigned', 'Standard', '0', '0.03125', '-16', '-16', '15.9688'; 'ACCTgtObjCntAlive', '392', '12', 'BE', 'unsigned', 'Standard', '0', '17', '0', '0', '65536'; 'ACCTgtObjDx', '272', '12', 'BE', 'unsigned', 'Standard', '0', '0.0625', '0', '0', '255.9375'; 'ACCTgtObjDy', '328', '11', 'BE', 'unsigned', 'Standard', '0', '0.125', '-128', '-128', '127.875'; 'ACCTgtObjExist', '338', '6', 'BE', 'unsigned', 'Standard', '0', '0.015625', '0', '0', '0.98438'; 'ACCTgtObjID', '312', '8', 'BE', 'unsigned', 'Standard', '0', '1', '0', '0', '255'; 'ACCTgtObjObstcl', '323', '5', 'BE', 'unsigned', 'Standard', '0', '0.03125', '0', '0', '0.96875'; 'ACCTgtObjState', '389', '3', 'BE', 'unsigned', 'Standard', '0', '1', '0', '0', '7'; 'ACCTgtObjVideoCfmd', '388', '1', 'BE', 'unsigned', 'Standard', '0', '1', '0', '0', '1'; 'ACCTgtObjVx', '364', '12', 'BE', 'unsigned', 'Standard', '0', '0.0625', '-128', '-128', '127'; 'ACCTgtObjVy', '344', '10', 'BE', 'unsigned', 'Standard', '0', '0.125', '-64', '-64', '63.875'; 'ACC_DataRecReq', '485', '3', 'BE', 'unsigned', 'Standard', '0', '1', '0', '0', '7'; 'ACC_SOSReq', '483', '2', 'BE', 'unsigned', 'Standard', '0', '1', '0', '0', '3'; 'BrdgDst', '474', '6', 'BE', 'unsigned', 'Standard', '0', '10', '0', '0', '600'; 'CurveDst', '458', '6', 'BE', 'unsigned', 'Standard', '0', '10', '0', '0', '600'; 'DrvgOnHiWay', '408', '2', 'BE', 'unsigned', 'Standard', '0', '1', '0', '0', '3'; 'DrvgOnRiLane', '464', '2', 'BE', 'unsigned', 'Standard', '0', '1', '0', '0', '3'; 'DrvrSts', '492', '3', 'BE', 'unsigned', 'Standard', '0', '1', '0', '0', '7'; 'HandsoffDetd', '410', '2', 'BE', 'unsigned', 'Standard', '0', '1', '0', '0', '3'; 'MapDataValid', '495', '1', 'BE', 'unsigned', 'Standard', '0', '1', '0', '0', '1'; 'NavSpdLimUnit', '456', '2', 'BE', 'unsigned', 'Standard', '0', '1', '0', '0', '3'; 'RampDst', '440', '6', 'BE', 'unsigned', 'Standard', '0', '10', '0', '0', '600'; 'RoadCrvt', '430', '10', 'BE', 'unsigned', 'Standard', '0', '0.00032', '-0.16352', '-0.16352', '0.16352'; 'RoadCrvtFar', '446', '10', 'BE', 'unsigned', 'Standard', '0', '0.00032', '-0.16352', '-0.16352', '0.16352'; 'SpdLimit', '448', '8', 'BE', 'unsigned', 'Standard', '0', '1', '0', '0', '255'; 'SpdLimitDst', '424', '6', 'BE', 'unsigned', 'Standard', '0', '10', '0', '0', '600'; 'TunnelDst', '466', '6', 'BE', 'unsigned', 'Standard', '0', '10', '0', '0', '600' }
      settings: SourceProductBaseCode=VN  DataFormat=manually specified signals
  CheckSum8Bclc1 : MATLAB Function  TreatAsAtomicUnit=on
  CheckSum8Bclc2 : MATLAB Function  TreatAsAtomicUnit=on
  CheckSum8Bclc3 : MATLAB Function  TreatAsAtomicUnit=on
  CheckSum8Bclc4 : MATLAB Function  TreatAsAtomicUnit=on
  Constant : Constant  Value=0  OutDataTypeStr=Inherit: Inherit via back propagation
  Constant1 : Constant  Value=[0x53 0x00]  OutDataTypeStr=uint8
  Constant2 : Constant  Value=[0x00 0x00;0x54 0x00;0x55 0x00;0xc8 0x00;0x00 0x00;0x00 0x00;0x00 0x00;0x00 0x00]  OutDataTypeStr=uint8
  Constant3 : Constant  Value=[0x00 0x00;0x56 0x00; 0x57 0x00; 0x6d 0x00; 0x58 0x00; 0x59 0x00;0x00 0x00;0x00 0x00]  OutDataTypeStr=uint8
  Constant4 : Constant  Value=[0x00 0x00;0x4f 0x00; 0x50 0x00;0x51 0x00;0x52 0x00;0x00 0x00;0x00 0x00;0x00 0x00]  OutDataTypeStr=uint8
  Constant5 : Constant  Value=0  OutDataTypeStr=Inherit: Inherit via back propagation
  Constant6 : Constant  Value=0  OutDataTypeStr=Bus:IDC_L3_FD1_MSG_BUS
  Constant7 : Constant  Value=P_BCM_TurnLmpType
  Counter Limited : simulink/Sources/Counter Limited  uplimit=15  tsamp=-1
  HMA : Subsystem  Commented=on
  HMI : Subsystem
  IfPlanbus1 : InportShadow  Port=10
  Subsystem : Subsystem
  Subsystem1 : Subsystem
  Switch : Switch  Criteria=u2 ~= 0
  rollingcounter 1 : Subsystem
  rollingcounter 2 : Subsystem
  rollingcounter 3 : Subsystem
  rollingcounter 4 : Subsystem
  IFC_FD1 : Outport
  IFC_FD2 : Outport  Port=2
  IFC_FD3 : Outport  Port=3
  IFC_FD5 : Outport  Port=4
  IFC_FD6 : Outport  Port=5
  ACC_FD1 : Outport  Port=6
  ACC_FD2 : Outport  Port=7
  ACC_FD3 : Outport  Port=8
  IDC_L3_FD1 : Outport  Port=9
  wires:
  IfVCANBus/1 -> HMI/1(IfVCANBus), HMA/1(IfCANBus)
  IfVEQ4Bus/1 -> HMA/4(IfEQ4Bus)
  IfCALBus/1 -> HMA/2(IfCALBus)
  IfFaultTriggers/1 -> HMI/2(IfFaultTriggers), HMA/3(IfDIAGBus)
  IfLonCtrlBus/1 -> [IfLonCtrlBus], HMI/5(IfLonCtrlBus)
  IfOSMBus/1 -> HMI/6(IfOSMBus)
  IfAEBBus/1 -> HMI/7(IfAEBBus)
  IfEHRBus/1 -> HMI/8(IfEHRBus)
  IfDMSBus/1 -> HMI/9(IfDMSBus)
  LaneBus/1 -> HMI/10(LaneBus)
  RoadBus/1 -> HMI/11(RoadBus)
  Bus Selector2/1 -> Subsystem/4(IFCVirationWarning)  "<IFCVibrationWarning>"
  HMI/1(IfHMIBus) -> Bus Selector10/1, Bus Selector8/1, Bus Creator/1, Bus Selector6/1, Bus Selector5/1, Bus Selector19/1, Bus Selector3/1, Bus Selector2/1  "HMI"
  Bus Selector3/1 -> CAN FD Pack1/1  "<AESErrSts>"
  Bus Selector3/2 -> CAN FD Pack1/2  "<AESResp>"
  Bus Selector3/3 -> CAN FD Pack1/3  "<AESSts>"
  Bus Selector3/4 -> CAN FD Pack1/4  "<AESintervention>"
  Bus Selector3/5 -> CAN FD Pack1/5  "<CameraBlockageSts>"
  Bus Selector3/6 -> CAN FD Pack1/6  "<ELKMainState>"
  Bus Selector3/7 -> CAN FD Pack1/7  "<ELKResp>"
  Bus Selector3/8 -> CAN FD Pack1/8  "<ESSErrSts>"
  Bus Selector3/9 -> CAN FD Pack1/9  "<ESSSts>"
  Bus Selector3/10 -> CAN FD Pack1/10  "<ESS_PedResp>"
  Bus Selector3/11 -> CAN FD Pack1/11  "<ESS_VehResp>"
  Bus Selector3/12 -> CAN FD Pack1/12  "<ESSintervention>"
  Bus Selector3/13 -> CAN FD Pack1/13  "<IFCCalibrationSts>"
  Bus Selector3/14 -> CAN FD Pack1/14  "<IFCHUTInterface>"
  Bus Selector3/15 -> CAN FD Pack1/15  "<IFC_Handsoffwarn>"
  Bus Selector3/16 -> CAN FD Pack1/16  "<IFC_LaneCurve>"
  Bus Selector3/17 -> CAN FD Pack1/17  "<IFC_LeLaneTyp>"
  Bus Selector3/18 -> CAN FD Pack1/18  "<IFC_LeLane_dy>"
  Bus Selector3/19 -> CAN FD Pack1/19  "<IFC_NextLeLaneTyp>"
  Bus Selector3/20 -> CAN FD Pack1/20  "<IFC_NextLeLane_dy>"
  Bus Selector3/21 -> CAN FD Pack1/21  "<IFC_NextRiLaneTyp>"
  Bus Selector3/22 -> CAN FD Pack1/22  "<IFC_NextRiLane_dy>"
  Bus Selector3/23 -> CAN FD Pack1/23  "<IFC_RiLaneTyp>"
  Bus Selector3/24 -> CAN FD Pack1/24  "<IFC_RiLane_dy>"
  Bus Selector3/25 -> CAN FD Pack1/25  "<IntelligentEvaResp>"
  Bus Selector3/26 -> CAN FD Pack1/26  "<LCKResp>"
  Bus Selector3/27 -> CAN FD Pack1/27  "<LDWResp>"
  Bus Selector3/28 -> CAN FD Pack1/28  "<LDW_LKAWarn>"
  Bus Selector3/29 -> CAN FD Pack1/29  "<LDW_LKA_Snvty>"
  Bus Selector3/30 -> CAN FD Pack1/30  "<LKAResp>"
  Bus Selector3/31 -> CAN FD Pack1/31  "<LSSErrSts>"
  Bus Selector3/32 -> CAN FD Pack1/32  "<LSSFuncSts>"
  Bus Selector3/33 -> CAN FD Pack1/33  "<LSSIntervention>"
  Bus Selector3/34 -> CAN FD Pack1/34  "<LSSResp>"
  Bus Selector3/35 -> CAN FD Pack1/35  "<LSSWarnFormResp>"
  Bus Selector3/36 -> CAN FD Pack1/36  "<LaneAvailability>"
  Bus Selector3/37 -> CAN FD Pack1/41  "<TJA_FollowSts>"
  rollingcounter 1/1(cnt) -> CAN FD Pack1/40, CAN FD Pack1/37, CAN FD Pack1/38, CAN FD Pack1/39
  IfVSMBus/1 -> [IfVSMBus], HMI/4(IfVSMBus)
  [IfVSMBus] -> Bus Selector4/1
  Bus Selector5/1 -> CAN FD Pack3/1  "<IFC_Line01_Curv>"
  Bus Selector5/2 -> CAN FD Pack3/2  "<IFC_Line01_CurvChange>"
  Bus Selector5/3 -> CAN FD Pack3/3  "<IFC_Line01_Dy>"
  Bus Selector5/4 -> CAN FD Pack3/4  "<IFC_Line01_Type>"
  Bus Selector5/5 -> CAN FD Pack3/5  "<IFC_Line02_Curv>"
  Bus Selector5/6 -> CAN FD Pack3/6  "<IFC_Line02_CurvChange>"
  Bus Selector5/7 -> CAN FD Pack3/7  "<IFC_Line02_Dy>"
  Bus Selector5/8 -> CAN FD Pack3/8  "<IFC_Line02_Type>"
  Bus Selector5/9 -> CAN FD Pack3/9  "<IFC_Line03_Curv>"
  Bus Selector5/10 -> CAN FD Pack3/10  "<IFC_Line03_CurvChange>"
  Bus Selector5/11 -> CAN FD Pack3/11  "<IFC_Line03_Dy>"
  Bus Selector5/12 -> CAN FD Pack3/12  "<IFC_Line03_Type>"
  Bus Selector5/13 -> CAN FD Pack3/13  "<IFC_Line04_Curv>"
  Bus Selector5/14 -> CAN FD Pack3/14  "<IFC_Line04_CurvChange>"
  Bus Selector5/15 -> CAN FD Pack3/15  "<IFC_Line04_Dy>"
  Bus Selector5/16 -> CAN FD Pack3/16  "<IFC_Line04_Type>"
  Bus Selector5/17 -> CAN FD Pack3/17  "<IFC_Roadedge01_Curv>"
  Bus Selector5/18 -> CAN FD Pack3/18  "<IFC_Roadedge01_CurvChange>"
  Bus Selector5/19 -> CAN FD Pack3/19  "<IFC_Roadedge01_Dy>"
  Bus Selector5/20 -> CAN FD Pack3/20  "<IFC_Roadedge01_Type>"
  Bus Selector5/21 -> CAN FD Pack3/21  "<IFC_Roadedge02_Curv>"
  Bus Selector5/22 -> CAN FD Pack3/22  "<IFC_Roadedge02_CurvChange>"
  Bus Selector5/23 -> CAN FD Pack3/23  "<IFC_Roadedge02_Dy>"
  Bus Selector5/24 -> CAN FD Pack3/24  "<IFC_Roadedge02_Type>"
  Bus Selector6/1 -> CAN FD Pack4/3  "<IFC_Line01_HeadingAngle>"
  Bus Selector6/2 -> CAN FD Pack4/6  "<IFC_Line02_HeadingAngle>"
  Bus Selector6/3 -> CAN FD Pack4/9  "<IFC_Line03_HeadingAngle>"
  Bus Selector6/4 -> CAN FD Pack4/12  "<IFC_Line04_HeadingAngle>"
  Bus Selector6/5 -> CAN FD Pack4/15  "<IFC_Roadedge01_HeadingAngle>"
  Bus Selector6/6 -> CAN FD Pack4/18  "<IFC_Roadedge02_HeadingAngle>"
  Bus Selector7/1 -> CAN FD Pack6/1  "<ACC_CRInterface>"
  [IfLonCtrlBus] -> Bus Creator/2
  Bus Creator/1 -> Subsystem1/1(In13), Bus Selector9/1, Bus Selector7/1
  Bus Selector7/2 -> CAN FD Pack6/2  "<ActualTargetSpeed>"
  Bus Selector7/3 -> CAN FD Pack6/4  "<Longctrl_Decel_Req>"
  Bus Selector7/4 -> CAN FD Pack6/5  "<Longctrl_Decel_ReqValue>"
  Bus Selector7/5 -> CAN FD Pack6/6  "<Longctrl_DrvOFF_Req>"
  Bus Selector7/6 -> CAN FD Pack6/7  "<Longctrl_EngTrqReq>"
  Bus Selector7/7 -> CAN FD Pack6/8  "<Longctrl_EngTrqReqActive>"
  Bus Selector7/8 -> CAN FD Pack6/9  "<Longctrl_FuelCutOffPrevn>"
  Bus Selector7/11 -> CAN FD Pack6/12  "<Longctrl_ModSts>"
  Bus Selector7/12 -> CAN FD Pack6/13  "<Longctrl_ParkShiftReq>"
  Bus Selector7/13 -> CAN FD Pack6/14  "<Longctrl_VehHldReq>"
  Bus Selector8/1 -> CAN FD Pack5/1  "<ACC_EgoStatus>"
  Bus Selector8/2 -> CAN FD Pack5/2  "<ACC_FctSts>"
  Bus Selector8/3 -> CAN FD Pack5/3  "<ACC_InterSysInfoDisp>"
  Bus Selector8/4 -> CAN FD Pack5/4  "<ACC_LeTargrtDection>"
  Bus Selector8/5 -> CAN FD Pack5/5  "<ACC_LeTargrt_02_Detn>"
  Bus Selector8/6 -> CAN FD Pack5/6  "<ACC_LeTgtDx>"
  Bus Selector8/7 -> CAN FD Pack5/7  "<ACC_LeTgtDy>"
  Bus Selector8/8 -> CAN FD Pack5/8  "<ACC_LeTgtHeading>"
  Bus Selector10/1 -> CAN FD Pack7/1  "<ACCTgtObjAx>"
  Bus Selector10/2 -> CAN FD Pack7/2  "<ACCTgtObjAy>"
  Bus Selector10/3 -> CAN FD Pack7/3  "<ACCTgtObjCntAlive>"
  Bus Selector10/4 -> CAN FD Pack7/4  "<ACCTgtObjDx>"
  Bus Selector10/5 -> CAN FD Pack7/5  "<ACCTgtObjDy>"
  Bus Selector10/6 -> CAN FD Pack7/6  "<ACCTgtObjExist>"
  Bus Selector10/7 -> CAN FD Pack7/7  "<ACCTgtObjID>"
  Bus Selector10/8 -> CAN FD Pack7/8  "<ACCTgtObjObstcl>"
  Bus Selector10/9 -> CAN FD Pack7/9  "<ACCTgtObjState>"
  Bus Selector10/10 -> CAN FD Pack7/10  "<ACCTgtObjVideoCfmd>"
  Bus Selector10/11 -> CAN FD Pack7/11  "<ACCTgtObjVx>"
  Bus Selector10/12 -> CAN FD Pack7/12  "<ACCTgtObjVy>"
  Bus Selector10/13 -> CAN FD Pack7/14  "<ACC_SOSReq>"
  Bus Selector10/14 -> CAN FD Pack7/15  "<BrdgDst>"
  Bus Selector10/15 -> CAN FD Pack7/16  "<CurveDst>"
  Bus Selector10/16 -> CAN FD Pack7/17  "<DrvgOnHiWay>"
  Bus Selector10/17 -> CAN FD Pack7/18  "<DrvgOnRiLane>"
  Bus Selector10/18 -> CAN FD Pack7/19  "<DrvrSts>"
  Bus Selector10/19 -> CAN FD Pack7/20  "<HandsoffDetd>"
  Bus Selector10/20 -> CAN FD Pack7/21  "<MapDataValid>"
  Bus Selector10/21 -> CAN FD Pack7/22  "<NavSpdLimUnit>"
  Bus Selector10/22 -> CAN FD Pack7/23  "<RampDst>"
  Bus Selector10/23 -> CAN FD Pack7/24  "<RoadCrvt>"
  Bus Selector10/24 -> CAN FD Pack7/25  "<RoadCrvtFar>"
  Bus Selector10/25 -> CAN FD Pack7/26  "<SpdLimit>"
  Bus Selector10/26 -> CAN FD Pack7/27  "<SpdLimitDst>"
  Bus Selector10/27 -> CAN FD Pack7/28  "<TunnelDst>"
  rollingcounter 2/1(cnt) -> CAN FD Pack2/6
  Bus Selector4/10 -> CAN FD Pack2/16  "<TSRWarnResp>"
  Bus Selector4/9 -> CAN FD Pack2/15  "<TSRTrfcSignValCfdc>"
  Bus Selector4/11 -> CAN FD Pack2/17  "<TSR_Snvty>"
  Bus Selector4/8 -> CAN FD Pack2/14  "<TSRTrfcSignVal>"
  Bus Selector4/7 -> CAN FD Pack2/13  "<TSRSts>"
  Bus Selector4/6 -> CAN FD Pack2/12  "<TSRSpdLimWarn>"
  Bus Selector4/5 -> CAN FD Pack2/11  "<TSRSpdLimUnit>"
  Bus Selector4/4 -> CAN FD Pack2/10  "<TSRSpdLimSts>"
  Bus Selector4/3 -> CAN FD Pack2/9  "<TSRSpdLimCfdc>"
  Bus Selector4/2 -> CAN FD Pack2/8  "<TSRSpdLim>"
  Bus Selector4/1 -> CAN FD Pack2/7  "<TSRResp>"
  Bus Selector11/1 -> CheckSum8Bclc4/1(Data)  "<Data>"
  Constant4/1 -> CheckSum8Bclc4/2(DataID)
  CAN FD Pack1/1 -> Bus Selector11/1
  rollingcounter 3/1(cnt) -> CAN FD Pack6/15, CAN FD Pack6/16, CAN FD Pack6/17, CAN FD Pack6/18
  rollingcounter 4/1(cnt) -> CAN FD Pack5/77, CAN FD Pack5/76, CAN FD Pack5/75, CAN FD Pack5/74, CAN FD Pack5/73
  Subsystem/1(IFC_FD1_MsgByte) -> IFC_FD1/1
  CheckSum8Bclc4/1(MsgByte) -> IFC_FD2/1
  CAN FD Pack2/1 -> Bus Selector12/1
  Constant1/1 -> CheckSum8Bclc1/2(DataID)
  Bus Selector12/1 -> CheckSum8Bclc1/1(Data)  "<Data>"
  CheckSum8Bclc1/1(MsgByte) -> IFC_FD3/1
  CAN FD Pack3/1 -> Bus Selector13/1
  Bus Selector13/1 -> IFC_FD5/1  "<Data>"
  Bus Selector14/1 -> IFC_FD6/1  "<Data>"
  CAN FD Pack4/1 -> Bus Selector14/1
  Bus Selector15/1 -> CheckSum8Bclc2/1(Data)  "<Data>"
  Constant2/1 -> CheckSum8Bclc2/2(DataID)
  CAN FD Pack6/1 -> Bus Selector15/1
  Constant3/1 -> CheckSum8Bclc3/2(DataID)
  Bus Selector16/1 -> CheckSum8Bclc3/1(Data)  "<Data>"
  CAN FD Pack5/1 -> Bus Selector16/1
  Bus Selector17/1 -> ACC_FD3/1  "<Data>"
  CAN FD Pack7/1 -> Bus Selector17/1
  CheckSum8Bclc2/1(MsgByte) -> ACC_FD1/1
  CheckSum8Bclc3/1(MsgByte) -> ACC_FD2/1
  Subsystem1/1(Out9) -> ACC_FD1MSG/1
  IfPlanbus/1 -> HMI/3(IfPlanbus)
  IfPlanbus1/1 -> Bus Selector18/1
  Bus Selector18/1 -> Subsystem1/2(<PLAN_Longctrl_DecelToStopReq>), CAN FD Pack5/60, CAN FD Pack6/3  "<PLAN_Longctrl_DecelToStopReq>"
  Bus Selector8/9 -> CAN FD Pack5/9  "<ACC_LeTgtObjBarDisp>"
  Bus Selector8/10 -> CAN FD Pack5/10  "<ACC_LeTgtTyp>"
  Bus Selector8/11 -> CAN FD Pack5/11  "<ACC_LeTgt_02_Dy>"
  Bus Selector8/12 -> CAN FD Pack5/12  "<ACC_LeTgt_02_Dx>"
  Bus Selector8/13 -> CAN FD Pack5/13  "<ACC_LeTgt_02_Typ>"
  Bus Selector8/14 -> CAN FD Pack5/14  "<ACC_LeTgtfusion>"
  Bus Selector8/15 -> CAN FD Pack5/15  "<ACC_ModDisp>"
  Bus Selector8/16 -> CAN FD Pack5/16  "<ACC_ObjDetecte>"
  Bus Selector8/17 -> CAN FD Pack5/17  "<ACC_PotentialTgtDetn>"
  Bus Selector8/18 -> CAN FD Pack5/18  "<ACC_PotentialTgtDx>"
  Bus Selector8/19 -> CAN FD Pack5/19  "<ACC_PotentialTgtDy>"
  Bus Selector8/20 -> CAN FD Pack5/20  "<ACC_PotentialTgtHeading>"
  Bus Selector8/21 -> CAN FD Pack5/21  "<ACC_PotentialTgtTyp>"
  Bus Selector8/22 -> CAN FD Pack5/22  "<ACC_PotentialTgtfusion>"
  Bus Selector8/23 -> CAN FD Pack5/23  "<ACC_RiTargrtDetn>"
  Bus Selector8/24 -> CAN FD Pack5/24  "<ACC_RiTargrt_02_Detn>"
  Bus Selector8/25 -> CAN FD Pack5/25  "<ACC_RiTgtDx>"
  Bus Selector8/26 -> CAN FD Pack5/26  "<ACC_RiTgtDy>"
  Bus Selector8/27 -> CAN FD Pack5/27  "<ACC_RiTgtHeading>"
  Bus Selector8/28 -> CAN FD Pack5/28  "<ACC_RiTgtObjBarDisp>"
  Bus Selector8/29 -> CAN FD Pack5/29  "<ACC_RiTgtTyp>"
  Bus Selector8/30 -> CAN FD Pack5/30  "<ACC_RiTgt_02_Dx>"
  Bus Selector8/31 -> CAN FD Pack5/31  "<ACC_RiTgt_02_Dy>"
  Bus Selector8/32 -> CAN FD Pack5/32  "<ACC_RiTgt_02_Typ>"
  Bus Selector8/33 -> CAN FD Pack5/33  "<ACC_RiTgtfusion>"
  Bus Selector8/34 -> CAN FD Pack5/34  "<ACC_RlvTgtDetn>"
  Bus Selector8/35 -> CAN FD Pack5/35  "<ACC_RlvTgtDx>"
  Bus Selector8/36 -> CAN FD Pack5/36  "<ACC_RlvTgtDy>"
  Bus Selector8/37 -> CAN FD Pack5/37  "<ACC_RlvTgtHeading>"
  Bus Selector8/38 -> CAN FD Pack5/38  "<ACC_RlvTgtTyp>"
  Bus Selector8/39 -> CAN FD Pack5/39  "<ACC_RlvTgtfusion>"
  Bus Selector8/40 -> CAN FD Pack5/40  "<ACC_SpdSetValue>"
  Bus Selector8/41 -> CAN FD Pack5/41  "<ACC_TakeOverReq>"
  Bus Selector8/43 -> CAN FD Pack5/43  "<ACC_TimeGapSet>"
  Bus Selector8/42 -> CAN FD Pack5/42  "<ACC_TgtObjBarDisp>"
  Bus Selector8/44 -> CAN FD Pack5/44  "<ADAS_DriverInloop_Monitor>"
  Bus Selector8/45 -> CAN FD Pack5/45  "<ALC_InterSysInfoDisp>"
  Bus Selector8/46 -> CAN FD Pack5/46  "<ALC_Resp>"
  Bus Selector8/47 -> CAN FD Pack5/47  "<CruCha_ModDisp>"
  Bus Selector8/48 -> CAN FD Pack5/48  "<CruChar_InterSysInfoDisp>"
  Bus Selector8/49 -> CAN FD Pack5/49  "<HWA_InterSysInfoDisp>"
  Bus Selector8/50 -> CAN FD Pack5/50  "<HWA_LaneChange>"
  Bus Selector8/51 -> CAN FD Pack5/51  "<HWA_LaneChangeReq>"
  Bus Selector8/52 -> CAN FD Pack5/52  "<HWA_ModDisp>"
  Bus Selector8/53 -> CAN FD Pack5/53  "<HWA_Resp>"
  Bus Selector8/54 -> CAN FD Pack5/54  "<HWA_SnvtySet_Resp>"
  Bus Selector8/55 -> CAN FD Pack5/55  "<HWA_warning>"
  Bus Selector8/56 -> CAN FD Pack5/56  "<ICA_HandsOffResp>"
  Bus Selector8/57 -> CAN FD Pack5/57  "<ISL_InterSysInfoDisp>"
  Bus Selector8/58 -> CAN FD Pack5/58  "<ISL_Resp>"
  Bus Selector8/59 -> CAN FD Pack5/59  "<IntelligentCurveAct>"
  Bus Selector9/1 -> CAN FD Pack5/61  "<Longctrl_Decel_ReqValue>"
  Bus Selector9/2 -> CAN FD Pack5/62  "<Longctrl_Decel_Req>"
  Bus Selector9/3 -> CAN FD Pack5/63  "<Longctrl_DrvOFF_Req>"
  Bus Selector9/4 -> CAN FD Pack5/64  "<Longctrl_EngTrqReqActive>"
  Bus Selector9/5 -> CAN FD Pack5/65  "<Longctrl_EngTrqReq>"
  Bus Selector9/6 -> CAN FD Pack5/68  "<Longctrl_HazActv>"
  Bus Selector9/7 -> CAN FD Pack5/69  "<Longctrl_ModSts_DVR>"
  Bus Selector9/8 -> CAN FD Pack5/70  "<Longctrl_ParkShiftReq_DVR>"
  Bus Selector9/9 -> CAN FD Pack5/71  "<Longctrl_VehHldReq_DVR>"
  Bus Selector9/10 -> CAN FD Pack5/72  "<Request_driveoff>"
  Bus Selector9/11 -> CAN FD Pack5/78  "<TJA_ACC_SelSts>"
  Bus Selector9/12 -> CAN FD Pack5/79  "<TJA_ICA_InterSysInfoDisp>"
  Bus Selector9/13 -> CAN FD Pack5/80  "<TJA_ICA_ModDisp>"
  Bus Selector19/3 -> Switch/3  "<IDC_L2_TurnLightReq>"
  Bus Selector19/2 -> CAN FD Pack2/4  "<IDC_L2_FWiperReq>"
  Bus Selector19/1 -> CAN FD Pack2/3  "<IDC_L2_EmgyLightReq>"
  Bus Selector7/9 -> CAN FD Pack6/10  "<Longctrl_HCUTrqReq>"
  Bus Selector7/10 -> CAN FD Pack6/11  "<Longctrl_HCUTrqReqActive>"
  Constant5/1 -> Subsystem/3(IFCTrqOvlCMdReqValue)
  Constant/1 -> Subsystem/2(IFCFuncTrqCmdReqFlag)
  Constant6/1 -> Bus Assignment/1
  Bus Assignment/1 -> IDC_L3_FD1/1
  Counter Limited/1 -> Bus Assignment/5, Bus Assignment/4, Bus Assignment/3, Bus Assignment/2
  IfLatCtrlBus/1 -> Subsystem/1(IfLatCtrlBus)
  CSASim_IDC_L2_LampReq/1 -> Switch/1
  Constant7/1 -> Switch/2
  Switch/1 -> CAN FD Pack2/5
